simulink model "SimModel_7"  (R2016b)
settings: Solver=ode1  StartTime=0.00001  StopTime=1000  FixedStep=0.01  RelTol=1e-3
libraries: simulink x1
settings Model: Creator=Maksim  LastModifiedBy=Maksim

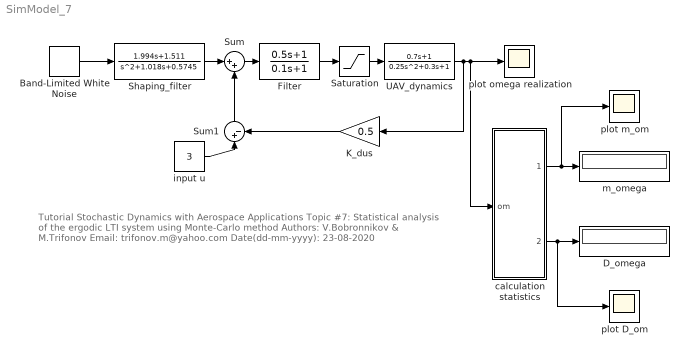
== system SimModel_7 ==
  note: Tutorial Stochastic Dynamics with Aerospace Applications
      | Topic #7: Statistical analysis of the ergodic LTI system using Monte-Carlo method
      | Authors: V.Bobronnikov & M.Trifonov
      | Email: trifonov.m@yahoo.com
      | Date(dd-mm-yyyy): 23-08-2020
  Band-Limited White Noise : simulink/Sources/Band-Limited White Noise  Cov=[1]  Ts=0.01  seed=[23551]
  D_omega : Display
  Filter : TransferFcn  Numerator=[0.5 1]  Denominator=[0.1 1]
  K_dus : Gain  Gain=0.5
  Saturation : Saturate  UpperLimit=2.5  LowerLimit=-2.5
  Shaping_filter : TransferFcn  Numerator=[1.994 1.511]  Denominator=[1 1.018 0.5745]
  Sum : Sum  Inputs=|++
  Sum1 : Sum  Inputs=|+-
  UAV_dynamics : TransferFcn  Numerator=[0.7 1]  Denominator=[0.25 0.3 1]
  calculation statistics : Subsystem
  input u : Constant  Value=3
  m_omega : Display
  plot omega realization : Scope
  plot D_om : Scope
  plot m_om : Scope
  wires:
  Filter/1 -> Saturation/1
  Sum/1 -> Filter/1
  Saturation/1 -> UAV_dynamics/1
  Band-Limited White Noise/1 -> Shaping_filter/1
  Shaping_filter/1 -> Sum/1
  K_dus/1 -> Sum1/2
  Sum1/1 -> Sum/2
  input u/1 -> Sum1/1
  UAV_dynamics/1 -> plot omega realization/1, calculation statistics/1(om), K_dus/1
  calculation statistics/1(m_om) -> plot m_om/1, m_omega/1
  calculation statistics/2(D_om) -> plot D_om/1, D_omega/1

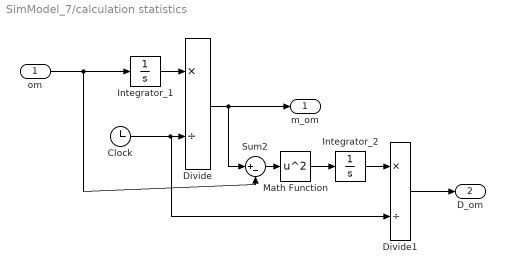
== system SimModel_7/calculation statistics ==
  om : Inport
  Clock : Clock
  Divide : Product  Inputs=*/
  Divide1 : Product  Inputs=*/
  Integrator_1 : Integrator
  Integrator_2 : Integrator
  Math Function : Math  Operator=square  SaturateOnIntegerOverflow=on
  Sum2 : Sum  Inputs=|+-
  m_om : Outport
  D_om : Outport  Port=2
  wires:
  om/1 -> Integrator_1/1, Sum2/2
  Integrator_1/1 -> Divide/1
  Clock/1 -> Divide1/2, Divide/2
  Divide/1 -> m_om/1, Sum2/1
  Divide1/1 -> D_om/1
  Math Function/1 -> Integrator_2/1
  Sum2/1 -> Math Function/1
  Integrator_2/1 -> Divide1/1
